simulink model "AOS_with_ACC__CM6"  (Simulink 9.1)
settings: Solver=ode45  StartTime=0.0  StopTime=inf  RelTol=1e-3  EnableMultiTasking=on
libraries: CarMaker4SL x59, simulink x10
(part 3 of 3)

== system AOS_with_ACC__CM6/CarMaker/VehicleControl/P_AOS/LCA/BlindSpotL/P_SwitchOff Simulation ==
  Sensor Index : Inport
  Constant1 : Constant
  Constant2 : Constant  Value=-1
  Constant3 : Constant  Value=0
  Relational Operator : RelationalOperator  Operator===  RndMeth=Simplest
  Stop Simulation : Stop
  Switch2 : Switch  Criteria=u2 > Threshold  SaturateOnIntegerOverflow=on
  wires:
  Constant1/1 -> Switch2/1
  Sensor Index/1 -> Relational Operator/1
  Constant3/1 -> Switch2/3
  Relational Operator/1 -> Switch2/2
  Constant2/1 -> Relational Operator/2
  Switch2/1 -> Stop Simulation/1

== system AOS_with_ACC__CM6/CarMaker/VehicleControl/P_AOS/LCA/FRSensor/P_SwitchOff Simulation ==
  Sensor Index : Inport
  Constant1 : Constant
  Constant2 : Constant  Value=-1
  Constant3 : Constant  Value=0
  Relational Operator : RelationalOperator  Operator===  RndMeth=Simplest
  Stop Simulation : Stop
  Switch2 : Switch  Criteria=u2 > Threshold  SaturateOnIntegerOverflow=on
  wires:
  Constant1/1 -> Switch2/1
  Sensor Index/1 -> Relational Operator/1
  Constant3/1 -> Switch2/3
  Relational Operator/1 -> Switch2/2
  Constant2/1 -> Relational Operator/2
  Switch2/1 -> Stop Simulation/1

== system AOS_with_ACC__CM6/CarMaker/VehicleControl/P_AOS/Predicted_ AOS_Condition/F_Left_sensor_OnComin_Vehicle/FLSensor ==
  note: Switch off simulation if LCA sensor not connected
  note: relevant target detected
  Bus Creator : BusCreator  Inputs=3
  Bus Selector : BusSelector  OutputSignals=relvTargetIndex,TargetDetected
  Bus Selector1 : BusSelector  OutputSignals=NearPnt ds_p,NearPnt dv_p
  Car ObjectSensor : CarMaker4SL/Car ObjectSensor  xname=RadarL
      settings: SourceProductName=CarMaker4SL
  Car ObjectSensor Object : CarMaker4SL/Car ObjectSensor Object  xname=INPORT  ximode=World Objects
      settings: SourceProductName=CarMaker4SL
  Ground : Ground
  No target : Constant  Value=-1
  P_SwitchOff Simulation : Subsystem
  Switch : Switch  Criteria=u2 > Threshold  SaturateOnIntegerOverflow=on
  Switch1 : Switch  Criteria=u2 > Threshold  SaturateOnIntegerOverflow=on
  Target dv : Constant  Value=-1
  Terminator{,1..6} (7 alike) : Terminator
  relevant  target : Outport
  wires:
  Switch/1 -> Bus Creator/2  "ds[m]"
  Bus Selector1/1 -> Switch/1  "<NearPnt ds_p>"
  No target/1 -> Switch/3
  Bus Selector1/2 -> Switch1/1  "<NearPnt dv_p>"
  Target dv/1 -> Switch1/3
  Switch1/1 -> Bus Creator/3  "dv[m/s]"
  Bus Creator/1 -> relevant  target/1
  Car ObjectSensor/1 -> P_SwitchOff Simulation/1(Sensor Index), Car ObjectSensor Object/1  "p_Sensor Index"
  Ground/1 -> Car ObjectSensor/1
  Car ObjectSensor/4 -> Bus Selector/1
  Bus Selector/2 -> Bus Creator/1, Switch1/2, Switch/2  "<TargetDetected>"
  Bus Selector/1 -> Car ObjectSensor Object/2  "<relvTargetIndex>"
  Car ObjectSensor Object/5 -> Bus Selector1/1
  Car ObjectSensor/2 -> Terminator/1
  Car ObjectSensor/3 -> Terminator1/1
  Car ObjectSensor Object/1 -> Terminator2/1
  Car ObjectSensor Object/2 -> Terminator3/1
  Car ObjectSensor Object/3 -> Terminator4/1
  Car ObjectSensor Object/4 -> Terminator5/1
  Car ObjectSensor Object/6 -> Terminator6/1

== system AOS_with_ACC__CM6/CarMaker/VehicleControl/AccelCtrl/ACC ECU/ACC Control/Distance Control Algorithm/desired ax ==
  note: desired ax =
  note: delta_ds
  Target.ds[m] : Inport
  Target.dv[m/s] : Inport  Port=2
  desired distance[m] : Inport  Port=3
  ax speed control : Inport  Port=4
  Add : Sum  SaturateOnIntegerOverflow=on  OutDataTypeStr=Inherit: Same as first input
  Divide : Product  Inputs=*/  SaturateOnIntegerOverflow=on  OutDataTypeStr=Inherit: Same as first input
  Divide1 : Product  Inputs=*/  SaturateOnIntegerOverflow=on  OutDataTypeStr=Inherit: Same as first input
  MinMax : MinMax  Inputs=2  SaturateOnIntegerOverflow=on  InputSameDT=on
  Read init distctrl.kd from Inf : CarMaker4SL/Read CM Parameter  xfile=Vehicle  xkey=AccelCtrl.ACC.DistCtrl.kd  xnout=1  xdefaults=36  xmuxed=off
      settings: SourceProductName=CarMaker4SL
  Read init distctrl.kv from Inf1 : CarMaker4SL/Read CM Parameter  xfile=Vehicle  xkey=AccelCtrl.ACC.DistCtrl.kv  xnout=1  xdefaults=2  xmuxed=off
      settings: SourceProductName=CarMaker4SL
  Subtract : Sum  Inputs=+-  SaturateOnIntegerOverflow=on  OutDataTypeStr=Inherit: Same as first input
  desired ax : Outport
  wires:
  MinMax/1 -> desired ax/1
  ax speed control/1 -> MinMax/2
  Add/1 -> MinMax/1
  Divide1/1 -> Add/2
  Divide/1 -> Add/1
  Subtract/1 -> Divide/1
  desired distance[m]/1 -> Subtract/2
  Target.ds[m]/1 -> Subtract/1
  Target.dv[m/s]/1 -> Divide1/1
  Read init distctrl.kd from Inf/1 -> Divide/2
  Read init distctrl.kv from Inf1/1 -> Divide1/2

== system AOS_with_ACC__CM6/CarMaker/VehicleControl/AccelCtrl/ACC ECU/ACC Control/Speed Control Algorithm/desired ax ==
  desire speed[m/s] : Inport
  Divide : Product  Inputs=*/  SaturateOnIntegerOverflow=on  OutDataTypeStr=Inherit: Same as first input
  Read Car.v[m/s] : CarMaker4SL/Read CM Dict  xname=Car.v  xsync=off
  Read init spdctrl.kv from Inf : CarMaker4SL/Read CM Parameter  xfile=Vehicle  xkey=AccelCtrl.ACC.SpdCtrl.kv  xnout=1  xdefaults=13  xmuxed=off
      settings: SourceProductName=CarMaker4SL
  Sum : Sum  Inputs=|+-  SaturateOnIntegerOverflow=on  OutDataTypeStr=Inherit: Same as first input
  desired ax : Outport
  wires:
  Divide/1 -> desired ax/1
  desire speed[m/s]/1 -> Sum/1
  Read Car.v[m/s]/1 -> Sum/2
  Sum/1 -> Divide/1
  Read init spdctrl.kv from Inf/1 -> Divide/2

== system AOS_with_ACC__CM6/CarMaker/VehicleControl/P_AOS/Predicted_ AOS_Condition/F_Left_sensor_OnComin_Vehicle/FLSensor/P_SwitchOff Simulation ==
  Sensor Index : Inport
  Constant1 : Constant
  Constant2 : Constant  Value=-1
  Constant3 : Constant  Value=0
  Relational Operator : RelationalOperator  Operator===  RndMeth=Simplest
  Stop Simulation : Stop
  Switch2 : Switch  Criteria=u2 > Threshold  SaturateOnIntegerOverflow=on
  wires:
  Constant1/1 -> Switch2/1
  Sensor Index/1 -> Relational Operator/1
  Constant3/1 -> Switch2/3
  Relational Operator/1 -> Switch2/2
  Constant2/1 -> Relational Operator/2
  Switch2/1 -> Stop Simulation/1

== stateflow chart CarMaker/VehicleControl/P_AOS/AOS_Ctrl/Simple_SteeringCtrl ==
  state SteerLeft
    SteerAngle = DMAngle
  state SteerMiddle
  state SteerRight
  state SteerMiddle2
  state IndicatorL
    L_Indic = 1
    Keep_On = 1
  state IndicatorR
    entry: R_Indic = 1
  state End
  note: Note: think of adapting the steering angle increment(0.01) to the speed of the velocity of the vehicle
  (default) -> IndicatorL
  SteerLeft -> SteerMiddle [order 1] : [carYpos == (L2Pos - factor)]{L_Indic = 0}
  SteerMiddle -> SteerMiddle [order 2] : [SteerAngle ~= 0 && after (50, msec) ]
      | {SteerAngle = SteerAngle - 0.01}
  SteerLeft -> SteerLeft [order 2] : [carYpos ~= (L2Pos - factor) && after (0.1, sec) ]
      | {SteerAngle = SteerAngle + 0.01}
  SteerMiddle -> IndicatorR [order 1] : [LCA == 3]
  IndicatorL -> SteerLeft : [after (3, sec)]
  IndicatorR -> SteerRight : [after (3,sec)]
  SteerMiddle2 -> SteerMiddle2 [order 1] : [SteerAngle ~= 0 && after (50, msec)]
      | {SteerAngle = SteerAngle + 0.01}
  SteerMiddle2 -> End [order 2] : [SteerAngle == 0]
      | {Keep_On = 0}
  SteerRight -> SteerRight [order 2] : [carYpos ~= (L1Pos - factor) && after (0.1, sec)]
      | {SteerAngle = SteerAngle - 0.01}
  SteerRight -> SteerMiddle2 [order 1] : [carYpos == L1Pos - factor ]
      | {R_Indic = 0}
  data: DMAngle input double; SteerAngle output double; carYpos input double; L2Pos input double; L1Pos input double; L_Indic output double; R_Indic output double; LCA input double; Keep_On output double; factor input double
